simulink model "hybrid_automata"  (R2019b)
settings: Solver=VariableStepAuto  StartTime=0.0  StopTime=10.0  FixedStep=0.1  RelTol=1e-3
libraries: simulink x2
settings Model: Creator=Isak  LastModifiedBy=Isak
settings SolverCC: ZeroCrossControl=EnableAll  ZeroCrossAlgorithm=Adaptive

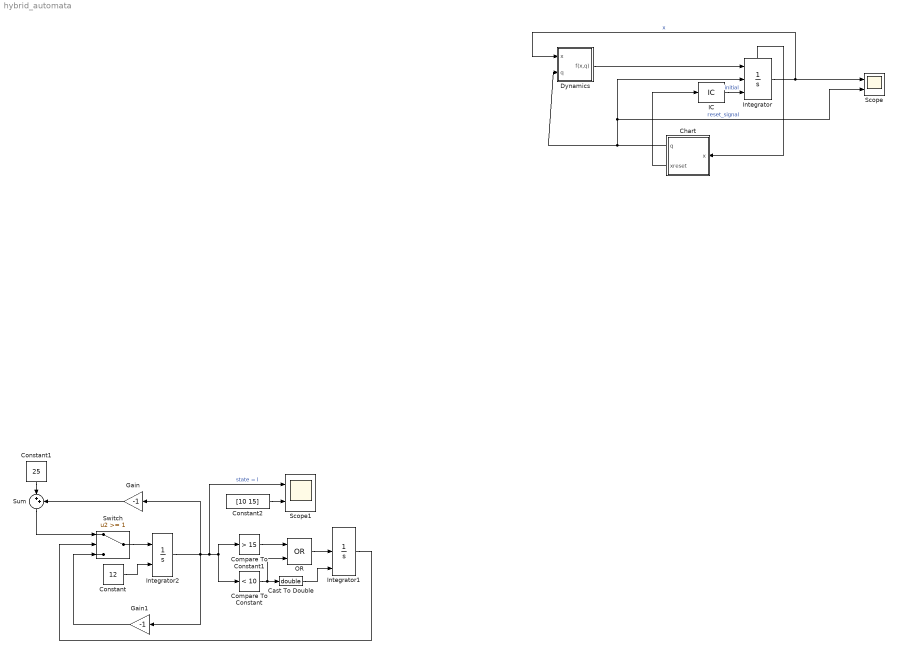
== system hybrid_automata ==
  Cast To Double : DataTypeConversion  OutDataTypeStr=double
  Chart : Stateflow chart  BlockKeywords=__PRM__SERIALIZED__DATA__:Stateflow Chart,Stateflow Diagram  TreatAsAtomicUnit=on
  Compare To Constant : simulink/Logic and Bit Operations/Compare To Constant  relop=<  const=10  OutDataTypeStr=boolean
  Compare To Constant1 : simulink/Logic and Bit Operations/Compare To Constant  relop=>  const=15  OutDataTypeStr=boolean
  Constant : Constant  Value=12
  Constant1 : Constant  Value=25
  Constant2 : Constant  Value=[10 15]
  Dynamics : Subsystem
  Gain : Gain  Gain=-1
  Gain1 : Gain  Gain=-1
  IC : InitialCondition  Value=[12;0]
  Integrator : Integrator  ExternalReset=rising  InitialConditionSource=external  InitialCondition=12  ShowStatePort=on
  Integrator1 : Integrator  ExternalReset=rising  InitialConditionSource=external
  Integrator2 : Integrator  InitialConditionSource=external  ZeroCross=off
  "OR " : Logic  Operator=OR  IconShape=distinctive  AllPortsSameDT=off  OutDataTypeStr=boolean
  Scope : Scope  NumInputPorts=2
  Scope1 : Scope  NumInputPorts=2
  Sum : Sum  Inputs=|++
  Switch : Switch  Threshold=1
  wires:
  IC/1 -> Integrator/3  "initial"
  Integrator/1 -> Dynamics/1(x), Scope/1  "x"
  Dynamics/1(f(x,q)) -> Integrator/1
  Chart/1(q) -> Scope/2, Integrator/2, Dynamics/2(q)  "reset_signal"
  Chart/2(xreset) -> IC/1
  Compare To Constant1/1 -> "OR "/1
  Compare To Constant/1 -> Cast To Double/1, "OR "/2
  Switch/1 -> Integrator2/1
  Constant/1 -> Integrator2/2
  Constant1/1 -> Sum/1
  Sum/1 -> Switch/1
  Gain/1 -> Sum/2
  Integrator2/1 -> Gain/1, Gain1/1, Scope1/1, Compare To Constant1/1, Compare To Constant/1  "state = l"
  Gain1/1 -> Switch/3
  Constant2/1 -> Scope1/2
  Cast To Double/1 -> Integrator1/3
  Integrator/State -> Chart/1(x)
  "OR "/1 -> Integrator1/2
  Integrator1/1 -> Switch/2

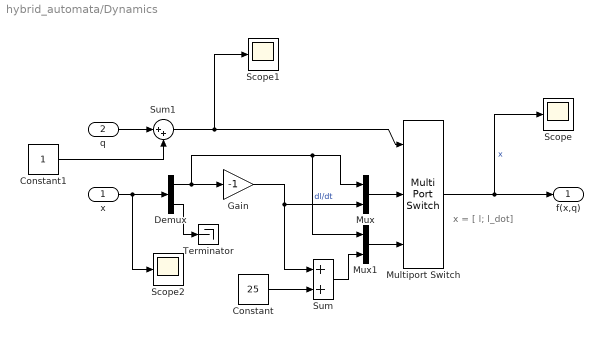
== system hybrid_automata/Dynamics ==
  note: x = [ l; l_dot]
  x : Inport
  q : Inport  Port=2
  Constant : Constant  Value=25
  Constant1 : Constant
  Demux : Demux  Outputs=2
  Gain : Gain  Gain=-1
  Multiport Switch : MultiPortSwitch  Inputs=2
  Mux : Mux  Inputs=2
  Mux1 : Mux  Inputs=2
  Scope : Scope
  Scope1 : Scope
  Scope2 : Scope
  Sum : Sum
  Sum1 : Sum  Inputs=|++
  Terminator : Terminator
  f(x,q) : Outport
  wires:
  Multiport Switch/1 -> Scope/1, f(x,q)/1  "x"
  Constant/1 -> Sum/2
  Sum1/1 -> Scope1/1, Multiport Switch/1
  q/1 -> Sum1/1
  Constant1/1 -> Sum1/2
  Mux/1 -> Multiport Switch/2
  Gain/1 -> Sum/1, Mux/2  "dl/dt"
  Mux1/1 -> Multiport Switch/3
  Sum/1 -> Mux1/2
  x/1 -> Scope2/1, Demux/1
  Demux/1 -> Mux1/1, Mux/1, Gain/1
  Demux/2 -> Terminator/1

== stateflow chart hybrid_automata/Chart ==
  state reset
    entry:
    xreset = [x(1);x(2)]
  state on
    entry:
    q=1;
  state off
    entry:
    q=0;
  (default) -> reset
  reset -> off : [true]
  off -> on : [x(1) < 10]/
      | {
      | xreset(1)=x(1);
      | xreset(2)=0
      | }
  on -> off : [x(1) < 15]{
      | xreset(1)=x(1);
      | xreset(2)=0;
      | }
  data: x input size=2; q output; xreset output size=2
